simulink model "VSM_specComp_DC"  (R2024b)
settings: Solver=ode3  StartTime=0.0  StopTime=4  FixedStep=HWSampleTime  RelTol=1e-3
PostLoadFcn:
  | EXEC_MODE=ExecutionMode.SIMULATION;
  | %Sim_TP33_VSM_HSS_init
InitFcn:
  | %EXEC_MODE=ExecutionMode.SIMULATION;
  | %Sim_TP33_VSM_HSS_init
StopFcn:
  | %sim2struct
undefined symbols (not defined in the file): ControlSampleTime, DiscIntNeverNeededParam, fault_dur, Grid, HWSampleTime, Ion, LCL, Lithium, Manage, Param, SM, t_fault, V_DC, VSMCTRL
libraries: FriedrichLibrary x76, simulink x32, TriphaseHardwaremodule x24, spsThreePhaseSeriesRLCBranchLib x8, spsThreePhaseVIMeasurementLib x8, spsThreePhaseBreakerLib x8, spsGroundLib x4, spsUniversalBridgeLib x4, spsVoltageMeasurementLib x4, spsEdgeDetectorLib x4, spsMeanLib x4, simulink_extras x4
(part 6 of 10)

== system VSM_specComp_DC/VSM_3/VSM1/VSM/CONTROL/Virtual Circuit1 ==
  Param : Inport
  Reset : Inport  Port=2
  i_dq0 : Inport  Port=3
  Phi : Inport  Port=4
  Bus Selector : BusSelector  OutputSignals=R1,L1
  Bus Selector1 : BusSelector  OutputSignals=R1t,tauR,L1t,tauL
  Current Predictor : Subsystem  Commented=on
  L_Matrix : Gain  Gain=[0 -1 0;1 0 0; 0 0 0]
  L_Matrix1 : Gain  Gain=[0 -1 0;1 0 0; 0 0 0]
  PT1 : Subsystem  mask{K=1, Init=0, Ts=ControlSampleTime}
      mask prompts: K "Gain"; Init "Initial input"; Ts "Sample time"
      mask DialogControl DescGroupVar Prompt: PT1 discrete
      mask DialogControl DescTextVar Prompt: Simple discrete PT1
      mask Display:
      | text(0.5,0.5,get_param(gcb,'K'),'HorizontalAlignment','center','VerticalAlignment','Bottom')
      | text(0.5,0.5,'1 + s.tau','HorizontalAlignment','center','VerticalAlignment','Top')
      | plot([0.3 0.7],[0.5 0.5])
  PT2 : Subsystem  Commented=on  mask{K=1, Init=0, Ts=ControlSampleTime}
      mask prompts: K "Gain"; Init "Initial input"; Ts "Sample time"
      mask DialogControl DescGroupVar Prompt: PT1 discrete
      mask DialogControl DescTextVar Prompt: Simple discrete PT1
      mask Display:
      | text(0.5,0.5,get_param(gcb,'K'),'HorizontalAlignment','center','VerticalAlignment','Bottom')
      | text(0.5,0.5,'1 + s.tau','HorizontalAlignment','center','VerticalAlignment','Top')
      | plot([0.3 0.7],[0.5 0.5])
  "Param " : InportShadow
  Phi1 : InportShadow  Port=4
  Product : Product  Multiplication=Matrix(*)
  Product1 : Product  Multiplication=Matrix(*)
  Product2 : Product  Commented=on  Multiplication=Matrix(*)
  Product3 : Product  Multiplication=Matrix(*)
  R_Matrix : Gain  Gain=[1 0 0;0 1 0; 0 0 0]
  R_Matrix1 : Gain  Gain=[1 0 0;0 1 0; 0 0 0]
  Reset1 : InportShadow  Port=2
  Scope : Scope  NumInputPorts=2
  Scope1 : Scope
  Sum : Sum  Inputs=++|
  Sum1 : Sum  Inputs=++|
  Sum2 : Sum  Inputs=|++
  " u_dq0" : Outport
  wires:
  Product3/1 -> Scope/1
  Reset1/1 -> PT2/3(Reset)
  Reset/1 -> PT1/3(Reset)
  Phi1/1 -> PT2/4(Phi)
  PT1/1(Y) -> Product1/2
  Sum2/1 -> " u_dq0"/1
  Sum1/1 -> Sum2/2
  Product2/1 -> Sum1/2, Scope1/1
  PT2/1(Y) -> Product2/2
  L_Matrix1/1 -> Product2/1
  Bus Selector1/3 -> L_Matrix1/1  "<L1t>"
  Bus Selector1/2 -> PT1/2(tau)  "<tauR>"
  Bus Selector1/4 -> PT2/2(tau)  "<tauL>"
  Bus Selector1/1 -> R_Matrix1/1  "<R1t>"
  Product1/1 -> Sum1/1, Scope/2
  R_Matrix1/1 -> Product1/1
  Product/1 -> Sum2/1
  "Param "/1 -> Bus Selector1/1
  Sum/1 -> Product/1
  R_Matrix/1 -> Sum/2, Product3/1
  L_Matrix/1 -> Sum/1
  Bus Selector/2 -> L_Matrix/1  "<L1>"
  i_dq0/1 -> Product/2, Product3/2, PT1/1(U), PT2/1(U)
  Bus Selector/1 -> R_Matrix/1  "<R1>"
  Param/1 -> Bus Selector/1

== system VSM_specComp_DC/VSM_3/VSM1/VSM/CONTROL/active_damping ==
  enable_damp_dq : Inport
  Reset : Inport  Port=2
  u_dq0 : Inport  Port=3
  Phi : Inport  Port=4
  Bus Selector : BusSelector  OutputSignals=Damp_dq,Damp_dq,Damp_CM,OmLead,OmLag
  Integrator (inertia) : DiscreteIntegrator  gainval=1  ExternalReset=rising  InitialConditionSource=external  InitialCondition=1  SampleTime=ControlSampleTime  ICPrevOutput=DiscIntNeverNeededParam  ICPrevScaledInput=DiscIntNeverNeededParam
  Mux : Mux  Inputs=3
  Product{,1..3} (4 alike) : Product
  Sum : Sum  Inputs=|+-
  Sum2 : Sum  Inputs=++|
  Unit Delay2 : UnitDelay  InitialCondition=[0 0 0]  SampleTime=ControlSampleTime  HasFrameUpgradeWarning=on
  dq0->ab0 phi : FriedrichLibrary/Transformations/dq0->ab0 phi  SystemSampleTime=-1  VariantActivationTime=update diagram  AllowFlexibleInterface=on  Latency=0  AutoFrameSizeCalculation=off
  damp_dq0 : Outport  VectorParamsAs1DForOutWhenUnconnected=off
  wires:
  Bus Selector/5 -> Product3/2  "<OmLag>"
  Bus Selector/4 -> Product2/1  "<OmLead>"
  dq0->ab0 phi/1 -> Integrator (inertia)/3
  Unit Delay2/1 -> dq0->ab0 phi/1
  Reset/1 -> Integrator (inertia)/2
  Phi/1 -> dq0->ab0 phi/2
  Product1/1 -> damp_dq0/1
  Mux/1 -> Product/1, Product1/1  "enable"
  Product/1 -> Product2/2, Sum2/1
  u_dq0/1 -> Product/2
  Bus Selector/3 -> Mux/3  "<Damp_CM>"
  Bus Selector/2 -> Mux/2  "<Damp_dq>"
  Bus Selector/1 -> Mux/1  "<Damp_dq>"
  enable_damp_dq/1 -> Bus Selector/1
  Sum/1 -> Integrator (inertia)/1
  Sum2/1 -> Product1/2, Product3/1
  Product3/1 -> Sum/2
  Integrator (inertia)/1 -> Sum2/2, Unit Delay2/1
  Product2/1 -> Sum/1

== system VSM_specComp_DC/VSM_3/VSM1/VSM/CONTROL/dq0 to duty ==
  phi_rad : Inport
  u_dq0 : Inport  Port=2
  u_dc : Inport  Port=3
  Bias : Bias  Bias=Ctrl.PWM.tauT*Ctrl.PU.omegab  SaturateOnIntegerOverflow=off
  Bus Creator3 : BusCreator  Inputs=2
  Divide : Product  Inputs=*/
  Gain : Gain  Gain=eye(NrChannels,3)  Multiplication=Matrix(K*u)
  Modulation : FriedrichLibrary/Transformations/Modulation  Method=Sine Modulation  Ts=ControlSampleTime
  SMA : FriedrichLibrary/Discrete Stuff/SMA  n_samples=1/ControlSampleTime/100  init_out=0
  Saturation : Saturate  UpperLimit=inf  LowerLimit=1
  Signal Specification1 : SignalSpecification
  dq0->ab0 phi : FriedrichLibrary/Transformations/dq0->ab0 phi  SystemSampleTime=-1  VariantActivationTime=update diagram  AllowFlexibleInterface=on  Latency=0  AutoFrameSizeCalculation=off
  d : Outport  VectorParamsAs1DForOutWhenUnconnected=off
  pwmDiag : Outport  Port=2  VectorParamsAs1DForOutWhenUnconnected=off
  wires:
  SMA/1 -> Divide/2
  Saturation/1 -> SMA/1
  Signal Specification1/1 -> d/1
  Gain/1 -> Signal Specification1/1, Bus Creator3/1  "pwm"
  Bus Creator3/1 -> pwmDiag/1  "pwmDiag"
  u_dc/1 -> Saturation/1
  Bias/1 -> dq0->ab0 phi/2
  Modulation/1 -> Gain/1
  dq0->ab0 phi/1 -> Divide/1
  Divide/1 -> Modulation/1  "ab0 norm"
  u_dq0/1 -> dq0->ab0 phi/1
  phi_rad/1 -> Bias/1, Bus Creator3/2  "phi"

== system VSM_specComp_DC/VSM_3/VSM1/VSM/CONTROL/i_dq_ctrl ==
  note: PI Control
  note: Outrouting
  note: Inrouting
  Param : Inport
  enable_cc : Inport  Port=2
  sp_cc : Inport  Port=3
  ms_i_inv_dq : Inport  Port=4
  u_ff_dq : Inport  Port=5
  u_inv_dq : Inport  Port=6
  Enable : EnablePort  StatesWhenEnabling=reset
  Bus Creator2 : BusCreator  Inputs=4
  Bus Selector13 : BusSelector  OutputSignals=init_u_inv
  Constant : Constant
  Demux : Demux  Outputs=2
  From1 : From  Commented=on  GotoTag=initU
  Gain1 : Gain  Commented=on  Gain=Kff
  Gain2 : Gain  Gain=L_inv
  Gain4 : Gain  Gain=[0 -1;1 0]  Multiplication=Matrix(K*u)
  Gain5 : Gain  Commented=on  Gain=1-Kff
  Mux : Mux  Inputs=2
  PI : Subsystem
  Product : Product
  Product1 : Product
  Product2 : Product
  Scope : Scope  NumInputPorts=3
  Step : Step  Time=8  Before=1  After=0  SampleTime=0
  Sum1 : Sum  Inputs=+++
  Sum2 : Sum  Commented=on  Inputs=|+-
  Sum3 : Sum  Inputs=|+-
  Switch1 : Switch  Commented=on  Criteria=u2 > Threshold  SaturateOnIntegerOverflow=off  InputSameDT=off
  sp_u_inv_dq : Outport  VectorParamsAs1DForOutWhenUnconnected=off
  CCdiag : Outport  Port=2  VectorParamsAs1DForOutWhenUnconnected=off
  wires:
  PI/1(u) -> Sum1/1  "pi"
  Constant/1 -> Product1/2, Product2/2
  Demux/1 -> Product2/1
  Product2/1 -> Mux/1
  Product1/1 -> Mux/2
  Demux/2 -> Product1/1
  Mux/1 -> PI/1(di)
  ms_i_inv_dq/1 -> Gain4/1, Sum3/2, [i_dq]
  Product/1 -> [sp_u_dq], sp_u_inv_dq/1
  Gain5/1 -> Switch1/3
  u_ff_dq/1 -> Gain5/1, Gain1/1, PI/2(u0), Scope/2
  [i_dq] -> Bus Creator2/2  "i_dq"
  [sp_i_dq] -> Bus Creator2/1  "sp_i_dq"
  Bus Creator2/1 -> CCdiag/1
  [Enable] -> Bus Creator2/4  "enable_cc"
  enable_cc/1 -> [Enable]  "enable_cc"
  [sp_u_dq] -> Bus Creator2/3  "sp_u_dq"
  [Enable] -> Product/1
  Bus Selector13/1 -> [initU]  "<init_u_inv>"
  Param/1 -> Bus Selector13/1
  sp_cc/1 -> Sum3/1, [sp_i_dq]
  Sum3/1 -> Demux/1
  [Enable] -> PI/Enable
  u_inv_dq/1 -> Switch1/1
  Sum1/1 -> Product/2, Scope/1
  From1/1 -> Switch1/2
  Gain2/1 -> Sum2/2  "dq decouple"
  Gain4/1 -> Gain2/1
  Switch1/1 -> Sum2/1

== system VSM_specComp_DC/VSM_3/VSM1/VSM/MANAGEMENT/Subsystem1 ==
  In1 : Inport
  <i_inv_dq0> : Inport  Port=2
  <u_cap_ab0> : Inport  Port=3
  <PQ_out> : Inport  Port=4
  enable : Inport  Port=5
  "AL brechen AL nicht mit FCN lösbar " : Memory
  Add2 : Sum  Inputs=+-
  Constant : Constant
  Divide : Product  Inputs=*/
  Math Function1 : Math  Operator=square  SignedPower=on
  Math Function2 : Math  Operator=square  SignedPower=on
  Selector2 : Selector  InputPortWidth=3  IndexOptions=Index vector (dialog)  Indices=[1 2]  OutputSizes=1
  Sqrt1 : Sqrt
  Sqrt2 : Sqrt
  Subsystem : Subsystem
  Subsystem1 : Subsystem
  Sum of Elements1 : Sum  Inputs=+
  Sum of Elements2 : Sum  Inputs=+
  CC : Outport
  sp_CC : Outport  Port=2
  wires:
  Subsystem1/2(i_abs_pre) -> Subsystem/6(i abs_pre)
  Add2/1 -> Subsystem1/Enable
  enable/1 -> Subsystem/Enable, Add2/2
  Constant/1 -> Add2/1
  Divide/1 -> Subsystem1/1(In1)
  Subsystem1/1(i_pq_pre) -> Subsystem/5(PQ_pre)
  <PQ_out>/1 -> Subsystem/2(PQ_out), Divide/1
  Subsystem/2(CC) -> CC/1
  In1/1 -> Math Function1/1
  Subsystem/1(i_sp) -> sp_CC/1  "sp_CC"
  <i_inv_dq0>/1 -> "AL brechen AL nicht mit FCN lösbar "/1
  <u_cap_ab0>/1 -> Selector2/1
  Math Function2/1 -> Sum of Elements2/1
  Sqrt1/1 -> Subsystem/4(U_cap), Divide/2
  "AL brechen AL nicht mit FCN lösbar "/1 -> Subsystem/1(i_inv)
  Sum of Elements2/1 -> Sqrt1/1
  Sqrt2/1 -> Subsystem1/2(In2), Subsystem/3(iabs)
  Math Function1/1 -> Sum of Elements1/1
  Selector2/1 -> Math Function2/1
  Sum of Elements1/1 -> Sqrt2/1

== system VSM_specComp_DC/VSM_3/VSM1/VSM/MANAGEMENT/current_watchdog ==
  |i| set : Inport
  |i| reset : Inport  Port=2
  i_ab : Inport  Port=3
  sp_gain : Inport  Port=4
  PQ : Inport  Port=5
  i_inv : Inport  Port=6
  active_current_watchdog : EnablePort  StatesWhenEnabling=reset
  Divide : Product  Inputs=/**
  MATLAB Function : MATLAB Function  Commented=on  TreatAsAtomicUnit=on
  Math Function1 : Math  Operator=square  SignedPower=on
  Math Function2 : Math  Operator=square  SignedPower=on
  Math Function3 : Math  Operator=square  SignedPower=on
  Relational Operator : RelationalOperator  Operator=<=  OutDataTypeStr=boolean  InputSameDT=off
  Relational Operator1 : RelationalOperator  Operator=<=  OutDataTypeStr=boolean  InputSameDT=off
  S-R Flip-Flop1 : simulink_extras/Flip Flops/S-R Flip-Flop  initial_condition=0
  Scope : Scope  NumInputPorts=3
  Scope1 : Scope
  Sum of Elements1 : Sum  Inputs=+
  Terminator1 : Terminator
  enable_cc : Outport  VectorParamsAs1DForOutWhenUnconnected=off
  sp_gain_wd : Outport  Port=2  VectorParamsAs1DForOutWhenUnconnected=off
  wires:
  i_inv/1 -> MATLAB Function/4(i_inv)
  PQ/1 -> MATLAB Function/3(p), Scope1/1
  MATLAB Function/2(i) -> sp_gain_wd/1
  MATLAB Function/1(CC) -> Scope/1, enable_cc/1
  sp_gain/1 -> Divide/3
  |i| set/1 -> Math Function2/1, Divide/1
  |i| reset/1 -> Math Function3/1, Divide/2
  Math Function3/1 -> Relational Operator1/2
  S-R Flip-Flop1/2 -> Terminator1/1
  Relational Operator1/1 -> S-R Flip-Flop1/2
  Math Function1/1 -> Sum of Elements1/1
  Sum of Elements1/1 -> Relational Operator/2, MATLAB Function/1(abs), Relational Operator1/1
  i_ab/1 -> Math Function1/1
  Math Function2/1 -> MATLAB Function/2(set), Relational Operator/1

== system VSM_specComp_DC/VSM_3/VSM1/VSM/MANAGEMENT/sp_VSM ==
  EnableRateLimit : Inport
  CMD : Inport  Port=2
  MEAS : Inport  Port=3
  Bus Creator : BusCreator  Inputs=3
  Bus Selector1 : BusSelector  OutputSignals=u_out.u_out_ab0
  Bus Selector6 : BusSelector  OutputSignals=Param.VSM.sp_f,Param.VSM.sp_E,Param.VSM.sp_PQ,Param.VSM.sp_PQ_limit
  "CMD " : InportShadow  Port=2
  E(PQ) : Subsystem
  PQ(U) Limit : Subsystem
  RateLimit : Subsystem
  Saturation : Saturate  UpperLimit=1  LowerLimit=-1
  sp_VSM : Outport  VectorParamsAs1DForOutWhenUnconnected=off
  wires:
  Saturation/1 -> RateLimit/1(PQ)
  "CMD "/1 -> E(PQ)/2(cmd)
  Bus Creator/1 -> sp_VSM/1
  Bus Selector6/1 -> Bus Creator/1  "<sp_f>"
  MEAS/1 -> Bus Selector1/1
  CMD/1 -> Bus Selector6/1
  PQ(U) Limit/1(sp_PQ_limit) -> Bus Creator/3  "sp_PQ"
  Bus Selector6/4 -> PQ(U) Limit/2(enable)  "<sp_PQ_limit>"
  Bus Selector1/1 -> PQ(U) Limit/3(u_out)  "<u_out_ab0>"
  RateLimit/1(PQslow) -> PQ(U) Limit/1(sp_PQ), E(PQ)/3(sp_PQ)
  EnableRateLimit/1 -> RateLimit/Enable  "ENABLED"
  Bus Selector6/3 -> Saturation/1  "<sp_PQ>"
  Bus Selector6/2 -> E(PQ)/1(E)  "<sp_E>"
  E(PQ)/1(sp_E) -> Bus Creator/2  "sp_E"

== system VSM_specComp_DC/VSM_3/VSM1/VSM/Meas/SI -> pu ==
  MeasIn : Inport
  Bus Creator1 : BusCreator  Inputs=5
  Bus Selector : BusSelector  OutputSignals=meas_u_out,meas_i_out,meas_i_inverter,meas_u_dc,meas_u_cap
  Normalize : Gain  Gain=1/PU.Ub  OutDataTypeStr=double  RndMeth=Round
  Normalize1 : Gain  Gain=1/PU.Ib  OutDataTypeStr=double  RndMeth=Round
  Normalize2 : Gain  Gain=1/PU.Ib  OutDataTypeStr=double  RndMeth=Round
  Normalize3 : Gain  Gain=1/PU.Ub  OutDataTypeStr=double  RndMeth=Round
  Normalize4 : Gain  Gain=1/PU.Ub/2  OutDataTypeStr=double  RndMeth=Round
  MeasOut : Outport  VectorParamsAs1DForOutWhenUnconnected=off
  wires:
  MeasIn/1 -> Bus Selector/1
  Normalize/1 -> Bus Creator1/1  "meas_u_out"
  Normalize1/1 -> Bus Creator1/3  "meas_i_inverter"
  Normalize2/1 -> Bus Creator1/2  "meas_i_out"
  Normalize4/1 -> Bus Creator1/4  "meas_vol_dc"
  Bus Creator1/1 -> MeasOut/1
  Bus Selector/1 -> Normalize/1  "<meas_u_out>"
  Bus Selector/2 -> Normalize2/1  "<meas_i_out>"
  Bus Selector/3 -> Normalize1/1  "<meas_i_inverter>"
  Bus Selector/4 -> Normalize4/1  "<meas_u_dc>"
  Bus Selector/5 -> Normalize3/1  "<meas_u_cap>"
  Normalize3/1 -> Bus Creator1/5  "meas_u_cap"

== system VSM_specComp_DC/VSM_3/VSM1/VSM/Meas/meas_i_inv ==
  abc : Inport
  phi : Inport  Port=2
  Bus Creator1 : BusCreator  Inputs=3
  PhN->ab2 : FriedrichLibrary/Transformations/PhN->ab0  SystemSampleTime=-1  VariantActivationTime=update diagram  AllowFlexibleInterface=on  Latency=0  AutoFrameSizeCalculation=off
  ab0->dq0-faster : FriedrichLibrary/Transformations/ab0->dq0-faster  SystemSampleTime=-1  VariantActivationTime=update diagram  AllowFlexibleInterface=on  Latency=0  AutoFrameSizeCalculation=off
  i_inv_x : Outport  VectorParamsAs1DForOutWhenUnconnected=off
  wires:
  Bus Creator1/1 -> i_inv_x/1
  phi/1 -> ab0->dq0-faster/2
  abc/1 -> PhN->ab2/1, Bus Creator1/1  "i_inv_abc"
  PhN->ab2/1 -> ab0->dq0-faster/1, Bus Creator1/2  "i_inv_ab0"
  ab0->dq0-faster/1 -> Bus Creator1/3  "i_inv_dq0"

== system VSM_specComp_DC/VSM_3/VSM1/VSM/Meas/meas_i_out ==
  abc : Inport
  phi : Inport  Port=2
  Bus Creator1 : BusCreator  Inputs=3
  PhN->ab2 : FriedrichLibrary/Transformations/PhN->ab0  SystemSampleTime=-1  VariantActivationTime=update diagram  AllowFlexibleInterface=on  Latency=0  AutoFrameSizeCalculation=off
  ab0->dq0-faster : FriedrichLibrary/Transformations/ab0->dq0-faster  SystemSampleTime=-1  VariantActivationTime=update diagram  AllowFlexibleInterface=on  Latency=0  AutoFrameSizeCalculation=off
  i_out_x : Outport  VectorParamsAs1DForOutWhenUnconnected=off
  wires:
  Bus Creator1/1 -> i_out_x/1
  phi/1 -> ab0->dq0-faster/2
  abc/1 -> PhN->ab2/1, Bus Creator1/1  "i_out_abc"
  PhN->ab2/1 -> ab0->dq0-faster/1, Bus Creator1/2  "i_out_ab0"
  ab0->dq0-faster/1 -> Bus Creator1/3  "i_out_dq0"

== system VSM_specComp_DC/VSM_3/VSM1/VSM/Meas/meas_u_cap ==
  abc : Inport
  phi : Inport  Port=2
  Bus Creator1 : BusCreator  Inputs=3
  PhN->ab2 : FriedrichLibrary/Transformations/PhN->ab0  SystemSampleTime=-1  VariantActivationTime=update diagram  AllowFlexibleInterface=on  Latency=0  AutoFrameSizeCalculation=off
  ab0->dq0-faster : FriedrichLibrary/Transformations/ab0->dq0-faster  SystemSampleTime=-1  VariantActivationTime=update diagram  AllowFlexibleInterface=on  Latency=0  AutoFrameSizeCalculation=off
  u_cap_x : Outport  VectorParamsAs1DForOutWhenUnconnected=off
  wires:
  ab0->dq0-faster/1 -> Bus Creator1/3  "u_cap_dq0"
  PhN->ab2/1 -> Bus Creator1/2, ab0->dq0-faster/1  "u_cap_ab0"
  abc/1 -> Bus Creator1/1, PhN->ab2/1  "u_cap_abc"
  phi/1 -> ab0->dq0-faster/2
  Bus Creator1/1 -> u_cap_x/1

== system VSM_specComp_DC/VSM_3/VSM1/VSM/Meas/meas_u_out ==
  abc : Inport
  phi : Inport  Port=2
  Bus Creator1 : BusCreator  Inputs=3
  PhN->ab2 : FriedrichLibrary/Transformations/PhN->ab0  SystemSampleTime=-1  VariantActivationTime=update diagram  AllowFlexibleInterface=on  Latency=0  AutoFrameSizeCalculation=off
  ab0->dq0-faster : FriedrichLibrary/Transformations/ab0->dq0-faster  SystemSampleTime=-1  VariantActivationTime=update diagram  AllowFlexibleInterface=on  Latency=0  AutoFrameSizeCalculation=off
  u_out_x : Outport  VectorParamsAs1DForOutWhenUnconnected=off
  wires:
  ab0->dq0-faster/1 -> Bus Creator1/3  "u_out_dq0"
  PhN->ab2/1 -> Bus Creator1/2, ab0->dq0-faster/1  "u_out_ab0"
  abc/1 -> Bus Creator1/1, PhN->ab2/1  "u_out_abc"
  phi/1 -> ab0->dq0-faster/2
  Bus Creator1/1 -> u_out_x/1

== system VSM_specComp_DC/VSM_3/VSM1/command_center/cmd_VSM/Current Control ==
  note: else: init with u cap
  Bus Creator6 : BusCreator  Inputs=5
  Bus Creator7 : BusCreator  Inputs=3
  Init with u_inv [0/1] : Constant  Value=VSMCTRL.CC.init_uinv
  activate : Constant  Value=VSMCTRL.CC.activate
  external_stop_cc1 : Constant  Value=0
  external_stop_cc4 : Constant  Value=0
  i_reset_abs : Constant  Value=VSMCTRL.CC.i_reset
  i_set_abs : Constant  Value=VSMCTRL.CC.i_set
  i_sp_gain : Constant  Value=VSMCTRL.CC.i_sp_gain
  Current Control : Outport  VectorParamsAs1DForOutWhenUnconnected=off
  wires:
  Bus Creator6/1 -> Current Control/1  "CC"
  Init with u_inv [0/1]/1 -> Bus Creator6/1  "init_u_inv"
  external_stop_cc1/1 -> Bus Creator6/3  "ex_stop_cc"
  i_sp_gain/1 -> Bus Creator6/4  "i_sp_gain"
  i_set_abs/1 -> Bus Creator7/2  "abs_i_set"
  external_stop_cc4/1 -> Bus Creator6/2  "ex_start_cc"
  Bus Creator7/1 -> Bus Creator6/5  "watchdog"
  i_reset_abs/1 -> Bus Creator7/3  "abs_i_reset"
  activate/1 -> Bus Creator7/1  "activate"

== system VSM_specComp_DC/VSM_3/VSM1/command_center/cmd_VSM/Damping ==
  Bus Creator5 : BusCreator  Inputs=4
  EnableDamp_CM [0/1] : Constant  Value=VSMCTRL.VTFF.EnableCM
  EnableDamp_dq [0/1] : Constant  Value=VSMCTRL.VTFF.EnableDQ
  Omega Lag : Constant  Value=VSMCTRL.VTFF.OmLag
  Omega Lead : Constant  Value=VSMCTRL.VTFF.OmLead
  Damping : Outport  VectorParamsAs1DForOutWhenUnconnected=off
  wires:
  Omega Lag/1 -> Bus Creator5/4  "OmLag"
  Omega Lead/1 -> Bus Creator5/3  "OmLead"
  Bus Creator5/1 -> Damping/1
  EnableDamp_dq [0/1]/1 -> Bus Creator5/1  "Damp_dq"
  EnableDamp_CM [0/1]/1 -> Bus Creator5/2  "Damp_CM"

== system VSM_specComp_DC/VSM_3/VSM1/command_center/cmd_VSM/Manage ==
  Bus Creator : BusCreator  Inputs=2
  connect : Constant
  enable : Constant
  Manage : Outport  VectorParamsAs1DForOutWhenUnconnected=off
  wires:
  enable/1 -> Bus Creator/2  "enable"
  connect/1 -> Bus Creator/1  "connect"
  Bus Creator/1 -> Manage/1

== system VSM_specComp_DC/VSM_3/VSM1/command_center/cmd_VSM/Virtual Circuit ==
  Bus Creator9 : BusCreator  Inputs=7
  Virtual L1 : Constant  Value=VSMCTRL.VC.L1
  Virtual L1t : Constant  Value=VSMCTRL.VC.L1t
  Virtual R1 : Constant  Value=VSMCTRL.VC.R1
  Virtual R1t : Constant  Value=VSMCTRL.VC.R1t
  tau HP Slow : Constant  Value=VSMCTRL.VC.tauSlow
  tau Virtual L1 : Constant  Value=VSMCTRL.VC.tauL
  tau Virtual R1 : Constant  Value=VSMCTRL.VC.tauR
  Virtual Circuit : Outport  VectorParamsAs1DForOutWhenUnconnected=off
  wires:
  tau HP Slow/1 -> Bus Creator9/7  "tauS"
  tau Virtual L1/1 -> Bus Creator9/6  "tauL"
  tau Virtual R1/1 -> Bus Creator9/5  "tauR"
  Virtual L1/1 -> Bus Creator9/3  "L1"
  Bus Creator9/1 -> Virtual Circuit/1
  Virtual L1t/1 -> Bus Creator9/4  "L1t"
  Virtual R1t/1 -> Bus Creator9/2  "R1t"
  Virtual R1/1 -> Bus Creator9/1  "R1"

== system VSM_specComp_DC/VSM_3/VSM1/command_center/cmd_VSM/Virtual Synchronous Machine ==
  note: 0 Dekaktiviert Init Tiefpass
  note: 0 Dekaktiviert Init Tiefpass
  Bus Creator3 : BusCreator  Inputs=12
  E(sp_PQ) : Constant  Value=VSMCTRL.SP.E_comp
  Ta : Constant  Value=VSMCTRL.VSM.Ta
  Ta1 : Constant  Value=VSMCTRL.VSM.kpf
  Ta2 : Constant  Value=VSMCTRL.VSM.kdf
  Ta3 : Constant  Value=VSMCTRL.VSM.ku
  Ta4 : Constant  Value=VSMCTRL.VSM.Tu
  Ta5 : Constant  Value=0
  Ta6 : Constant  Value=0
  sp_E [pu] : Constant  Value=VSMCTRL.SP.E
  sp_PQ [pu] : Constant  Value=VSMCTRL.SP.PQ
  sp_PQ(U) limit : Constant  Value=VSMCTRL.SP.PQU_lim
  sp_f [Hz] : Constant  Value=VSMCTRL.SP.f
  Virtual Synchronous Machine : Outport  VectorParamsAs1DForOutWhenUnconnected=off
  wires:
  E(sp_PQ)/1 -> Bus Creator3/12  "sp_E_comp"
  Ta5/1 -> Bus Creator3/6  "Tuinit"
  Ta6/1 -> Bus Creator3/7  "TPinit"
  Ta1/1 -> Bus Creator3/2  "kpf"
  Ta2/1 -> Bus Creator3/3  "kdf"
  Ta3/1 -> Bus Creator3/4  "ku"
  Ta4/1 -> Bus Creator3/5  "Tu"
  Bus Creator3/1 -> Virtual Synchronous Machine/1
  Ta/1 -> Bus Creator3/1  "Ta"
  sp_PQ(U) limit/1 -> Bus Creator3/11  "sp_PQ_limit"
  sp_f [Hz]/1 -> Bus Creator3/8  "sp_f"
  sp_PQ [pu]/1 -> Bus Creator3/9  "sp_PQ"
  sp_E [pu]/1 -> Bus Creator3/10  "sp_E"

== system VSM_specComp_DC/VSM_4/VSM1/VSM/CONTROL/Subsystem1 ==
  <R1> : Inport
  <L1> : Inport  Port=2
  I : Inport  Port=3
  U_i : Inport  Port=4
  Enable : EnablePort
  MATLAB Function : MATLAB Function  TreatAsAtomicUnit=on
  Selector : Selector  InputPortWidth=3  IndexOptions=Index vector (dialog)  Indices=[1 2]  OutputSizes=1
  Selector1 : Selector  InputPortWidth=3  IndexOptions=Index vector (dialog)  Indices=[1 2]  OutputSizes=1
  phi_vsm : Outport
  U_v : Outport  Port=2
  wires:
  MATLAB Function/2(U_v) -> U_v/1
  MATLAB Function/1(phi_vsm) -> phi_vsm/1
  U_i/1 -> Selector1/1
  I/1 -> Selector/1
  Selector1/1 -> MATLAB Function/4(U_i)
  Selector/1 -> MATLAB Function/1(I)
  <R1>/1 -> MATLAB Function/3(R1)
  <L1>/1 -> MATLAB Function/2(L1)

== system VSM_specComp_DC/VSM_4/VSM1/VSM/CONTROL/VSMOC1 ==
  Manage : Inport
  Meas : Inport  Port=2
  u_inv_dq : Inport  Port=3
  Bus Selector1 : BusSelector  OutputSignals=enable_VSM.enable_ctrl,Param.VSM,enable_VSM.enable_inertia,sp_VSM
  Bus Selector11 : BusSelector  OutputSignals=phi
  Bus Selector2 : BusSelector  OutputSignals=PQ,PLL,u_cap.u_cap_dq0
  Selector : Selector  InputPortWidth=3  IndexOptions=Index vector (dialog)  Indices=[1 2]  OutputSizes=1
  Switch : Switch  Criteria=u2 ~= 0  SaturateOnIntegerOverflow=off  InputSameDT=off
  VSMOC : Subsystem
  phi_rad : Outport  VectorParamsAs1DForOutWhenUnconnected=off
  sp_u_inv_dq : Outport  Port=2  InitialOutput=[1 0]  VectorParamsAs1DForOutWhenUnconnected=off
  VSMdiag : Outport  Port=3  VectorParamsAs1DForOutWhenUnconnected=off
  wires:
  Bus Selector11/1 -> Switch/3  "<phi>"
  VSMOC/1(phi_rad) -> Switch/1
  VSMOC/3(VSMdiag) -> VSMdiag/1
  VSMOC/2(sp_u_inv_dq) -> sp_u_inv_dq/1
  Switch/1 -> phi_rad/1
  Manage/1 -> Bus Selector1/1
  Bus Selector1/1 -> VSMOC/Enable, Switch/2  "<enable_ctrl>"
  Meas/1 -> Bus Selector2/1
  Bus Selector2/2 -> VSMOC/5(PLL), Bus Selector11/1  "<PLL>"
  Bus Selector1/2 -> VSMOC/1(Param)  "<VSM>"
  Bus Selector1/3 -> VSMOC/2(enable_inertia)  "<enable_inertia>"
  Bus Selector1/4 -> VSMOC/3(sp_VSM)  "<sp_VSM>"
  u_inv_dq/1 -> VSMOC/6(u_inv_dq)
  Bus Selector2/3 -> Selector/1  "<u_cap_dq0>"
  Selector/1 -> VSMOC/7(u_cap_dq1)
  Bus Selector2/1 -> VSMOC/4(PQ_meas)  "<PQ>"

== system VSM_specComp_DC/VSM_4/VSM1/VSM/CONTROL/Virtual Circuit mit R und L ==
  Param : Inport
  Reset : Inport  Port=2
  i_dq0 : Inport  Port=3
  Phi : Inport  Port=4
  Bus Selector : BusSelector  OutputSignals=R1,L1
  Bus Selector1 : BusSelector  OutputSignals=R1t,tauR,L1t,tauL
  Current Predictor : Subsystem  Commented=on
  L_Matrix : Gain  Gain=[0 -1 0;1 0 0; 0 0 0]
  L_Matrix1 : Gain  Gain=[0 -1 0;1 0 0; 0 0 0]
  PT1 : Subsystem  mask{K=1, Init=0, Ts=ControlSampleTime}
      mask prompts: K "Gain"; Init "Initial input"; Ts "Sample time"
      mask DialogControl DescGroupVar Prompt: PT1 discrete
      mask DialogControl DescTextVar Prompt: Simple discrete PT1
      mask Display:
      | text(0.5,0.5,get_param(gcb,'K'),'HorizontalAlignment','center','VerticalAlignment','Bottom')
      | text(0.5,0.5,'1 + s.tau','HorizontalAlignment','center','VerticalAlignment','Top')
      | plot([0.3 0.7],[0.5 0.5])
  PT2 : Subsystem  mask{K=1, Init=0, Ts=ControlSampleTime}
      mask prompts: K "Gain"; Init "Initial input"; Ts "Sample time"
      mask DialogControl DescGroupVar Prompt: PT1 discrete
      mask DialogControl DescTextVar Prompt: Simple discrete PT1
      mask Display:
      | text(0.5,0.5,get_param(gcb,'K'),'HorizontalAlignment','center','VerticalAlignment','Bottom')
      | text(0.5,0.5,'1 + s.tau','HorizontalAlignment','center','VerticalAlignment','Top')
      | plot([0.3 0.7],[0.5 0.5])
  "Param " : InportShadow
  Phi1 : InportShadow  Port=4
  Product : Product  Multiplication=Matrix(*)
  Product1 : Product  Multiplication=Matrix(*)
  Product2 : Product  Multiplication=Matrix(*)
  R_Matrix : Gain  Gain=[1 0 0;0 1 0; 0 0 0]
  R_Matrix1 : Gain  Gain=[1 0 0;0 1 0; 0 0 0]
  Reset1 : InportShadow  Port=2
  Sum : Sum  Inputs=++|
  Sum1 : Sum  Inputs=++|
  Sum2 : Sum  Inputs=|++
  " u_dq0" : Outport
  wires:
  Param/1 -> Bus Selector/1
  Bus Selector/1 -> R_Matrix/1  "<R1>"
  i_dq0/1 -> Product/2, PT2/1(U), PT1/1(U)
  Bus Selector/2 -> L_Matrix/1  "<L1>"
  L_Matrix/1 -> Sum/1
  R_Matrix/1 -> Sum/2
  Sum/1 -> Product/1
  "Param "/1 -> Bus Selector1/1
  R_Matrix1/1 -> Product1/1
  Product1/1 -> Sum1/1
  Bus Selector1/1 -> R_Matrix1/1  "<R1t>"
  Bus Selector1/4 -> PT2/2(tau)  "<tauL>"
  Bus Selector1/2 -> PT1/2(tau)  "<tauR>"
  Bus Selector1/3 -> L_Matrix1/1  "<L1t>"
  L_Matrix1/1 -> Product2/1
  Product2/1 -> Sum1/2
  Sum2/1 -> " u_dq0"/1
  PT1/1(Y) -> Product1/2
  Phi/1 -> PT1/4(Phi)
  Phi1/1 -> PT2/4(Phi)
  Reset/1 -> PT1/3(Reset)
  Reset1/1 -> PT2/3(Reset)
  PT2/1(Y) -> Product2/2
  Product/1 -> Sum2/1

== system VSM_specComp_DC/VSM_4/VSM1/VSM/CONTROL/Virtual Circuit1 ==
  Param : Inport
  Reset : Inport  Port=2
  i_dq0 : Inport  Port=3
  Phi : Inport  Port=4
  Bus Selector : BusSelector  OutputSignals=R1,L1
  Bus Selector1 : BusSelector  OutputSignals=R1t,tauR,L1t,tauL
  Current Predictor : Subsystem  Commented=on
  L_Matrix : Gain  Gain=[0 -1 0;1 0 0; 0 0 0]
  L_Matrix1 : Gain  Gain=[0 -1 0;1 0 0; 0 0 0]
  PT1 : Subsystem  mask{K=1, Init=0, Ts=ControlSampleTime}
      mask prompts: K "Gain"; Init "Initial input"; Ts "Sample time"
      mask DialogControl DescGroupVar Prompt: PT1 discrete
      mask DialogControl DescTextVar Prompt: Simple discrete PT1
      mask Display:
      | text(0.5,0.5,get_param(gcb,'K'),'HorizontalAlignment','center','VerticalAlignment','Bottom')
      | text(0.5,0.5,'1 + s.tau','HorizontalAlignment','center','VerticalAlignment','Top')
      | plot([0.3 0.7],[0.5 0.5])
  PT2 : Subsystem  Commented=on  mask{K=1, Init=0, Ts=ControlSampleTime}
      mask prompts: K "Gain"; Init "Initial input"; Ts "Sample time"
      mask DialogControl DescGroupVar Prompt: PT1 discrete
      mask DialogControl DescTextVar Prompt: Simple discrete PT1
      mask Display:
      | text(0.5,0.5,get_param(gcb,'K'),'HorizontalAlignment','center','VerticalAlignment','Bottom')
      | text(0.5,0.5,'1 + s.tau','HorizontalAlignment','center','VerticalAlignment','Top')
      | plot([0.3 0.7],[0.5 0.5])
  "Param " : InportShadow
  Phi1 : InportShadow  Port=4
  Product : Product  Multiplication=Matrix(*)
  Product1 : Product  Multiplication=Matrix(*)
  Product2 : Product  Commented=on  Multiplication=Matrix(*)
  Product3 : Product  Multiplication=Matrix(*)
  R_Matrix : Gain  Gain=[1 0 0;0 1 0; 0 0 0]
  R_Matrix1 : Gain  Gain=[1 0 0;0 1 0; 0 0 0]
  Reset1 : InportShadow  Port=2
  Scope : Scope  NumInputPorts=2
  Scope1 : Scope
  Sum : Sum  Inputs=++|
  Sum1 : Sum  Inputs=++|
  Sum2 : Sum  Inputs=|++
  " u_dq0" : Outport
  wires:
  Param/1 -> Bus Selector/1
  Bus Selector/1 -> R_Matrix/1  "<R1>"
  i_dq0/1 -> PT2/1(U), PT1/1(U), Product3/2, Product/2
  Bus Selector/2 -> L_Matrix/1  "<L1>"
  L_Matrix/1 -> Sum/1
  R_Matrix/1 -> Product3/1, Sum/2
  Sum/1 -> Product/1
  "Param "/1 -> Bus Selector1/1
  Product/1 -> Sum2/1
  R_Matrix1/1 -> Product1/1
  Product1/1 -> Scope/2, Sum1/1
  Bus Selector1/1 -> R_Matrix1/1  "<R1t>"
  Bus Selector1/4 -> PT2/2(tau)  "<tauL>"
  Bus Selector1/2 -> PT1/2(tau)  "<tauR>"
  Bus Selector1/3 -> L_Matrix1/1  "<L1t>"
  L_Matrix1/1 -> Product2/1
  PT2/1(Y) -> Product2/2
  Product2/1 -> Scope1/1, Sum1/2
  Sum1/1 -> Sum2/2
  Sum2/1 -> " u_dq0"/1
  PT1/1(Y) -> Product1/2
  Phi1/1 -> PT2/4(Phi)
  Reset/1 -> PT1/3(Reset)
  Reset1/1 -> PT2/3(Reset)
  Product3/1 -> Scope/1

== system VSM_specComp_DC/VSM_4/VSM1/VSM/CONTROL/active_damping ==
  enable_damp_dq : Inport
  Reset : Inport  Port=2
  u_dq0 : Inport  Port=3
  Phi : Inport  Port=4
  Bus Selector : BusSelector  OutputSignals=Damp_dq,Damp_dq,Damp_CM,OmLead,OmLag
  Integrator (inertia) : DiscreteIntegrator  gainval=1  ExternalReset=rising  InitialConditionSource=external  InitialCondition=1  SampleTime=ControlSampleTime  ICPrevOutput=DiscIntNeverNeededParam  ICPrevScaledInput=DiscIntNeverNeededParam
  Mux : Mux  Inputs=3
  Product{,1..3} (4 alike) : Product
  Sum : Sum  Inputs=|+-
  Sum2 : Sum  Inputs=++|
  Unit Delay2 : UnitDelay  InitialCondition=[0 0 0]  SampleTime=ControlSampleTime  HasFrameUpgradeWarning=on
  dq0->ab0 phi : FriedrichLibrary/Transformations/dq0->ab0 phi  SystemSampleTime=-1  VariantActivationTime=update diagram  AllowFlexibleInterface=on  Latency=0  AutoFrameSizeCalculation=off
  damp_dq0 : Outport  VectorParamsAs1DForOutWhenUnconnected=off
  wires:
  Product2/1 -> Sum/1
  Integrator (inertia)/1 -> Unit Delay2/1, Sum2/2
  Product3/1 -> Sum/2
  Sum2/1 -> Product3/1, Product1/2
  Sum/1 -> Integrator (inertia)/1
  enable_damp_dq/1 -> Bus Selector/1
  Bus Selector/1 -> Mux/1  "<Damp_dq>"
  Bus Selector/2 -> Mux/2  "<Damp_dq>"
  Bus Selector/3 -> Mux/3  "<Damp_CM>"
  u_dq0/1 -> Product/2
  Product/1 -> Sum2/1, Product2/2
  Mux/1 -> Product1/1, Product/1  "enable"
  Product1/1 -> damp_dq0/1
  Phi/1 -> dq0->ab0 phi/2
  Reset/1 -> Integrator (inertia)/2
  Unit Delay2/1 -> dq0->ab0 phi/1
  dq0->ab0 phi/1 -> Integrator (inertia)/3
  Bus Selector/4 -> Product2/1  "<OmLead>"
  Bus Selector/5 -> Product3/2  "<OmLag>"

== system VSM_specComp_DC/VSM_4/VSM1/VSM/CONTROL/dq0 to duty ==
  phi_rad : Inport
  u_dq0 : Inport  Port=2
  u_dc : Inport  Port=3
  Bias : Bias  Bias=Ctrl.PWM.tauT*Ctrl.PU.omegab  SaturateOnIntegerOverflow=off
  Bus Creator3 : BusCreator  Inputs=2
  Divide : Product  Inputs=*/
  Gain : Gain  Gain=eye(NrChannels,3)  Multiplication=Matrix(K*u)
  Modulation : FriedrichLibrary/Transformations/Modulation  Method=Sine Modulation  Ts=ControlSampleTime
  SMA : FriedrichLibrary/Discrete Stuff/SMA  n_samples=1/ControlSampleTime/100  init_out=0
  Saturation : Saturate  UpperLimit=inf  LowerLimit=1
  Signal Specification1 : SignalSpecification
  dq0->ab0 phi : FriedrichLibrary/Transformations/dq0->ab0 phi  SystemSampleTime=-1  VariantActivationTime=update diagram  AllowFlexibleInterface=on  Latency=0  AutoFrameSizeCalculation=off
  d : Outport  VectorParamsAs1DForOutWhenUnconnected=off
  pwmDiag : Outport  Port=2  VectorParamsAs1DForOutWhenUnconnected=off
  wires:
  phi_rad/1 -> Bus Creator3/2, Bias/1  "phi"
  u_dq0/1 -> dq0->ab0 phi/1
  Divide/1 -> Modulation/1  "ab0 norm"
  dq0->ab0 phi/1 -> Divide/1
  Modulation/1 -> Gain/1
  Bias/1 -> dq0->ab0 phi/2
  u_dc/1 -> Saturation/1
  Bus Creator3/1 -> pwmDiag/1  "pwmDiag"
  Gain/1 -> Bus Creator3/1, Signal Specification1/1  "pwm"
  Signal Specification1/1 -> d/1
  Saturation/1 -> SMA/1
  SMA/1 -> Divide/2

== system VSM_specComp_DC/VSM_4/VSM1/VSM/CONTROL/i_dq_ctrl ==
  note: Inrouting
  note: Outrouting
  note: PI Control
  Param : Inport
  enable_cc : Inport  Port=2
  sp_cc : Inport  Port=3
  ms_i_inv_dq : Inport  Port=4
  u_ff_dq : Inport  Port=5
  u_inv_dq : Inport  Port=6
  Enable : EnablePort  StatesWhenEnabling=reset
  Bus Creator2 : BusCreator  Inputs=4
  Bus Selector13 : BusSelector  OutputSignals=init_u_inv
  Constant : Constant
  Demux : Demux  Outputs=2
  From1 : From  Commented=on  GotoTag=initU
  Gain1 : Gain  Commented=on  Gain=Kff
  Gain2 : Gain  Gain=L_inv
  Gain4 : Gain  Gain=[0 -1;1 0]  Multiplication=Matrix(K*u)
  Gain5 : Gain  Commented=on  Gain=1-Kff
  Mux : Mux  Inputs=2
  PI : Subsystem
  Product : Product
  Product1 : Product
  Product2 : Product
  Scope : Scope  NumInputPorts=3
  Step : Step  Time=8  Before=1  After=0  SampleTime=0
  Sum1 : Sum  Inputs=+++
  Sum2 : Sum  Commented=on  Inputs=|+-
  Sum3 : Sum  Inputs=|+-
  Switch1 : Switch  Commented=on  Criteria=u2 > Threshold  SaturateOnIntegerOverflow=off  InputSameDT=off
  sp_u_inv_dq : Outport  VectorParamsAs1DForOutWhenUnconnected=off
  CCdiag : Outport  Port=2  VectorParamsAs1DForOutWhenUnconnected=off
  wires:
  Switch1/1 -> Sum2/1
  Gain4/1 -> Gain2/1
  Gain2/1 -> Sum2/2  "dq decouple"
  From1/1 -> Switch1/2
  Sum1/1 -> Scope/1, Product/2
  u_inv_dq/1 -> Switch1/1
  [Enable] -> PI/Enable
  Sum3/1 -> Demux/1
  sp_cc/1 -> [sp_i_dq], Sum3/1
  Param/1 -> Bus Selector13/1
  Bus Selector13/1 -> [initU]  "<init_u_inv>"
  [Enable] -> Product/1
  [sp_u_dq] -> Bus Creator2/3  "sp_u_dq"
  enable_cc/1 -> [Enable]  "enable_cc"
  [Enable] -> Bus Creator2/4  "enable_cc"
  Bus Creator2/1 -> CCdiag/1
  [sp_i_dq] -> Bus Creator2/1  "sp_i_dq"
  [i_dq] -> Bus Creator2/2  "i_dq"
  u_ff_dq/1 -> Scope/2, PI/2(u0), Gain1/1, Gain5/1
  Gain5/1 -> Switch1/3
  Product/1 -> sp_u_inv_dq/1, [sp_u_dq]
  ms_i_inv_dq/1 -> [i_dq], Sum3/2, Gain4/1
  Mux/1 -> PI/1(di)
  Demux/2 -> Product1/1
  Product1/1 -> Mux/2
  Product2/1 -> Mux/1
  Demux/1 -> Product2/1
  Constant/1 -> Product2/2, Product1/2
  PI/1(u) -> Sum1/1  "pi"

== system VSM_specComp_DC/VSM_4/VSM1/VSM/MANAGEMENT/Subsystem1 ==
  In1 : Inport
  <i_inv_dq0> : Inport  Port=2
  <u_cap_ab0> : Inport  Port=3
  <PQ_out> : Inport  Port=4
  enable : Inport  Port=5
  "AL brechen AL nicht mit FCN lösbar " : Memory
  Add2 : Sum  Inputs=+-
  Constant : Constant
  Divide : Product  Inputs=*/
  Math Function1 : Math  Operator=square  SignedPower=on
  Math Function2 : Math  Operator=square  SignedPower=on
  Selector2 : Selector  InputPortWidth=3  IndexOptions=Index vector (dialog)  Indices=[1 2]  OutputSizes=1
  Sqrt1 : Sqrt
  Sqrt2 : Sqrt
  Subsystem : Subsystem
  Subsystem1 : Subsystem
  Sum of Elements1 : Sum  Inputs=+
  Sum of Elements2 : Sum  Inputs=+
  CC : Outport
  sp_CC : Outport  Port=2
  wires:
  Sum of Elements1/1 -> Sqrt2/1
  Selector2/1 -> Math Function2/1
  Math Function1/1 -> Sum of Elements1/1
  Sqrt2/1 -> Subsystem/3(iabs), Subsystem1/2(In2)
  Sum of Elements2/1 -> Sqrt1/1
  "AL brechen AL nicht mit FCN lösbar "/1 -> Subsystem/1(i_inv)
  Sqrt1/1 -> Divide/2, Subsystem/4(U_cap)
  Math Function2/1 -> Sum of Elements2/1
  <u_cap_ab0>/1 -> Selector2/1
  <i_inv_dq0>/1 -> "AL brechen AL nicht mit FCN lösbar "/1
  Subsystem/1(i_sp) -> sp_CC/1  "sp_CC"
  In1/1 -> Math Function1/1
  Subsystem/2(CC) -> CC/1
  <PQ_out>/1 -> Divide/1, Subsystem/2(PQ_out)
  Subsystem1/1(i_pq_pre) -> Subsystem/5(PQ_pre)
  Divide/1 -> Subsystem1/1(In1)
  Constant/1 -> Add2/1
  enable/1 -> Add2/2, Subsystem/Enable
  Add2/1 -> Subsystem1/Enable
  Subsystem1/2(i_abs_pre) -> Subsystem/6(i abs_pre)

== system VSM_specComp_DC/VSM_4/VSM1/VSM/MANAGEMENT/current_watchdog ==
  |i| set : Inport
  |i| reset : Inport  Port=2
  i_ab : Inport  Port=3
  sp_gain : Inport  Port=4
  PQ : Inport  Port=5
  i_inv : Inport  Port=6
  active_current_watchdog : EnablePort  StatesWhenEnabling=reset
  Divide : Product  Inputs=/**
  MATLAB Function : MATLAB Function  Commented=on  TreatAsAtomicUnit=on
  Math Function1 : Math  Operator=square  SignedPower=on
  Math Function2 : Math  Operator=square  SignedPower=on
  Math Function3 : Math  Operator=square  SignedPower=on
  Relational Operator : RelationalOperator  Operator=<=  OutDataTypeStr=boolean  InputSameDT=off
  Relational Operator1 : RelationalOperator  Operator=<=  OutDataTypeStr=boolean  InputSameDT=off
  S-R Flip-Flop1 : simulink_extras/Flip Flops/S-R Flip-Flop  initial_condition=0
  Scope : Scope  NumInputPorts=3
  Scope1 : Scope
  Sum of Elements1 : Sum  Inputs=+
  Terminator1 : Terminator
  enable_cc : Outport  VectorParamsAs1DForOutWhenUnconnected=off
  sp_gain_wd : Outport  Port=2  VectorParamsAs1DForOutWhenUnconnected=off
  wires:
  Math Function2/1 -> Relational Operator/1, MATLAB Function/2(set)
  i_ab/1 -> Math Function1/1
  Sum of Elements1/1 -> Relational Operator1/1, MATLAB Function/1(abs), Relational Operator/2
  Math Function1/1 -> Sum of Elements1/1
  Relational Operator1/1 -> S-R Flip-Flop1/2
  S-R Flip-Flop1/2 -> Terminator1/1
  Math Function3/1 -> Relational Operator1/2
  |i| reset/1 -> Divide/2, Math Function3/1
  |i| set/1 -> Divide/1, Math Function2/1
  sp_gain/1 -> Divide/3
  MATLAB Function/1(CC) -> enable_cc/1, Scope/1
  MATLAB Function/2(i) -> sp_gain_wd/1
  PQ/1 -> Scope1/1, MATLAB Function/3(p)
  i_inv/1 -> MATLAB Function/4(i_inv)

== system VSM_specComp_DC/VSM_4/VSM1/VSM/MANAGEMENT/sp_VSM ==
  EnableRateLimit : Inport
  CMD : Inport  Port=2
  MEAS : Inport  Port=3
  Bus Creator : BusCreator  Inputs=3
  Bus Selector1 : BusSelector  OutputSignals=u_out.u_out_ab0
  Bus Selector6 : BusSelector  OutputSignals=Param.VSM.sp_f,Param.VSM.sp_E,Param.VSM.sp_PQ,Param.VSM.sp_PQ_limit
  "CMD " : InportShadow  Port=2
  E(PQ) : Subsystem
  PQ(U) Limit : Subsystem
  RateLimit : Subsystem
  Saturation : Saturate  UpperLimit=1  LowerLimit=-1
  sp_VSM : Outport  VectorParamsAs1DForOutWhenUnconnected=off
  wires:
  E(PQ)/1(sp_E) -> Bus Creator/2  "sp_E"
  Bus Selector6/2 -> E(PQ)/1(E)  "<sp_E>"
  Bus Selector6/3 -> Saturation/1  "<sp_PQ>"
  EnableRateLimit/1 -> RateLimit/Enable  "ENABLED"
  RateLimit/1(PQslow) -> E(PQ)/3(sp_PQ), PQ(U) Limit/1(sp_PQ)
  Bus Selector1/1 -> PQ(U) Limit/3(u_out)  "<u_out_ab0>"
  Bus Selector6/4 -> PQ(U) Limit/2(enable)  "<sp_PQ_limit>"
  PQ(U) Limit/1(sp_PQ_limit) -> Bus Creator/3  "sp_PQ"
  CMD/1 -> Bus Selector6/1
  MEAS/1 -> Bus Selector1/1
  Bus Selector6/1 -> Bus Creator/1  "<sp_f>"
  Bus Creator/1 -> sp_VSM/1
  "CMD "/1 -> E(PQ)/2(cmd)
  Saturation/1 -> RateLimit/1(PQ)

== system VSM_specComp_DC/VSM_4/VSM1/VSM/Meas/SI -> pu ==
  MeasIn : Inport
  Bus Creator1 : BusCreator  Inputs=5
  Bus Selector : BusSelector  OutputSignals=meas_u_out,meas_i_out,meas_i_inverter,meas_u_dc,meas_u_cap
  Normalize : Gain  Gain=1/PU.Ub  OutDataTypeStr=double  RndMeth=Round
  Normalize1 : Gain  Gain=1/PU.Ib  OutDataTypeStr=double  RndMeth=Round
  Normalize2 : Gain  Gain=1/PU.Ib  OutDataTypeStr=double  RndMeth=Round
  Normalize3 : Gain  Gain=1/PU.Ub  OutDataTypeStr=double  RndMeth=Round
  Normalize4 : Gain  Gain=1/PU.Ub/2  OutDataTypeStr=double  RndMeth=Round
  MeasOut : Outport  VectorParamsAs1DForOutWhenUnconnected=off
  wires:
  Normalize3/1 -> Bus Creator1/5  "meas_u_cap"
  Bus Selector/5 -> Normalize3/1  "<meas_u_cap>"
  Bus Selector/4 -> Normalize4/1  "<meas_u_dc>"
  Bus Selector/3 -> Normalize1/1  "<meas_i_inverter>"
  Bus Selector/2 -> Normalize2/1  "<meas_i_out>"
  Bus Selector/1 -> Normalize/1  "<meas_u_out>"
  Bus Creator1/1 -> MeasOut/1
  Normalize4/1 -> Bus Creator1/4  "meas_vol_dc"
  Normalize2/1 -> Bus Creator1/2  "meas_i_out"
  Normalize1/1 -> Bus Creator1/3  "meas_i_inverter"
  Normalize/1 -> Bus Creator1/1  "meas_u_out"
  MeasIn/1 -> Bus Selector/1

== system VSM_specComp_DC/VSM_4/VSM1/VSM/Meas/meas_i_inv ==
  abc : Inport
  phi : Inport  Port=2
  Bus Creator1 : BusCreator  Inputs=3
  PhN->ab2 : FriedrichLibrary/Transformations/PhN->ab0  SystemSampleTime=-1  VariantActivationTime=update diagram  AllowFlexibleInterface=on  Latency=0  AutoFrameSizeCalculation=off
  ab0->dq0-faster : FriedrichLibrary/Transformations/ab0->dq0-faster  SystemSampleTime=-1  VariantActivationTime=update diagram  AllowFlexibleInterface=on  Latency=0  AutoFrameSizeCalculation=off
  i_inv_x : Outport  VectorParamsAs1DForOutWhenUnconnected=off
  wires:
  ab0->dq0-faster/1 -> Bus Creator1/3  "i_inv_dq0"
  PhN->ab2/1 -> Bus Creator1/2, ab0->dq0-faster/1  "i_inv_ab0"
  abc/1 -> Bus Creator1/1, PhN->ab2/1  "i_inv_abc"
  phi/1 -> ab0->dq0-faster/2
  Bus Creator1/1 -> i_inv_x/1

== system VSM_specComp_DC/VSM_4/VSM1/VSM/Meas/meas_i_out ==
  abc : Inport
  phi : Inport  Port=2
  Bus Creator1 : BusCreator  Inputs=3
  PhN->ab2 : FriedrichLibrary/Transformations/PhN->ab0  SystemSampleTime=-1  VariantActivationTime=update diagram  AllowFlexibleInterface=on  Latency=0  AutoFrameSizeCalculation=off
  ab0->dq0-faster : FriedrichLibrary/Transformations/ab0->dq0-faster  SystemSampleTime=-1  VariantActivationTime=update diagram  AllowFlexibleInterface=on  Latency=0  AutoFrameSizeCalculation=off
  i_out_x : Outport  VectorParamsAs1DForOutWhenUnconnected=off
  wires:
  ab0->dq0-faster/1 -> Bus Creator1/3  "i_out_dq0"
  PhN->ab2/1 -> Bus Creator1/2, ab0->dq0-faster/1  "i_out_ab0"
  abc/1 -> Bus Creator1/1, PhN->ab2/1  "i_out_abc"
  phi/1 -> ab0->dq0-faster/2
  Bus Creator1/1 -> i_out_x/1

== system VSM_specComp_DC/VSM_4/VSM1/VSM/Meas/meas_u_cap ==
  abc : Inport
  phi : Inport  Port=2
  Bus Creator1 : BusCreator  Inputs=3
  PhN->ab2 : FriedrichLibrary/Transformations/PhN->ab0  SystemSampleTime=-1  VariantActivationTime=update diagram  AllowFlexibleInterface=on  Latency=0  AutoFrameSizeCalculation=off
  ab0->dq0-faster : FriedrichLibrary/Transformations/ab0->dq0-faster  SystemSampleTime=-1  VariantActivationTime=update diagram  AllowFlexibleInterface=on  Latency=0  AutoFrameSizeCalculation=off
  u_cap_x : Outport  VectorParamsAs1DForOutWhenUnconnected=off
  wires:
  Bus Creator1/1 -> u_cap_x/1
  phi/1 -> ab0->dq0-faster/2
  abc/1 -> PhN->ab2/1, Bus Creator1/1  "u_cap_abc"
  PhN->ab2/1 -> ab0->dq0-faster/1, Bus Creator1/2  "u_cap_ab0"
  ab0->dq0-faster/1 -> Bus Creator1/3  "u_cap_dq0"

== system VSM_specComp_DC/VSM_4/VSM1/VSM/Meas/meas_u_out ==
  abc : Inport
  phi : Inport  Port=2
  Bus Creator1 : BusCreator  Inputs=3
  PhN->ab2 : FriedrichLibrary/Transformations/PhN->ab0  SystemSampleTime=-1  VariantActivationTime=update diagram  AllowFlexibleInterface=on  Latency=0  AutoFrameSizeCalculation=off
  ab0->dq0-faster : FriedrichLibrary/Transformations/ab0->dq0-faster  SystemSampleTime=-1  VariantActivationTime=update diagram  AllowFlexibleInterface=on  Latency=0  AutoFrameSizeCalculation=off
  u_out_x : Outport  VectorParamsAs1DForOutWhenUnconnected=off
  wires:
  Bus Creator1/1 -> u_out_x/1
  phi/1 -> ab0->dq0-faster/2
  abc/1 -> PhN->ab2/1, Bus Creator1/1  "u_out_abc"
  PhN->ab2/1 -> ab0->dq0-faster/1, Bus Creator1/2  "u_out_ab0"
  ab0->dq0-faster/1 -> Bus Creator1/3  "u_out_dq0"

== system VSM_specComp_DC/VSM_4/VSM1/command_center/cmd_VSM/Current Control ==
  note: else: init with u cap
  Bus Creator6 : BusCreator  Inputs=5
  Bus Creator7 : BusCreator  Inputs=3
  Init with u_inv [0/1] : Constant  Value=VSMCTRL.CC.init_uinv
  activate : Constant  Value=VSMCTRL.CC.activate
  external_stop_cc1 : Constant  Value=0
  external_stop_cc4 : Constant  Value=0
  i_reset_abs : Constant  Value=VSMCTRL.CC.i_reset
  i_set_abs : Constant  Value=VSMCTRL.CC.i_set
  i_sp_gain : Constant  Value=VSMCTRL.CC.i_sp_gain
  Current Control : Outport  VectorParamsAs1DForOutWhenUnconnected=off
  wires:
  activate/1 -> Bus Creator7/1  "activate"
  i_reset_abs/1 -> Bus Creator7/3  "abs_i_reset"
  Bus Creator7/1 -> Bus Creator6/5  "watchdog"
  external_stop_cc4/1 -> Bus Creator6/2  "ex_start_cc"
  i_set_abs/1 -> Bus Creator7/2  "abs_i_set"
  i_sp_gain/1 -> Bus Creator6/4  "i_sp_gain"
  external_stop_cc1/1 -> Bus Creator6/3  "ex_stop_cc"
  Init with u_inv [0/1]/1 -> Bus Creator6/1  "init_u_inv"
  Bus Creator6/1 -> Current Control/1  "CC"

== system VSM_specComp_DC/VSM_4/VSM1/command_center/cmd_VSM/Damping ==
  Bus Creator5 : BusCreator  Inputs=4
  EnableDamp_CM [0/1] : Constant  Value=VSMCTRL.VTFF.EnableCM
  EnableDamp_dq [0/1] : Constant  Value=VSMCTRL.VTFF.EnableDQ
  Omega Lag : Constant  Value=VSMCTRL.VTFF.OmLag
  Omega Lead : Constant  Value=VSMCTRL.VTFF.OmLead
  Damping : Outport  VectorParamsAs1DForOutWhenUnconnected=off
  wires:
  EnableDamp_CM [0/1]/1 -> Bus Creator5/2  "Damp_CM"
  EnableDamp_dq [0/1]/1 -> Bus Creator5/1  "Damp_dq"
  Bus Creator5/1 -> Damping/1
  Omega Lead/1 -> Bus Creator5/3  "OmLead"
  Omega Lag/1 -> Bus Creator5/4  "OmLag"

== system VSM_specComp_DC/VSM_4/VSM1/command_center/cmd_VSM/Manage ==
  Bus Creator : BusCreator  Inputs=2
  connect : Constant
  enable : Constant
  Manage : Outport  VectorParamsAs1DForOutWhenUnconnected=off
  wires:
  Bus Creator/1 -> Manage/1
  connect/1 -> Bus Creator/1  "connect"
  enable/1 -> Bus Creator/2  "enable"

== system VSM_specComp_DC/VSM_4/VSM1/command_center/cmd_VSM/Virtual Circuit ==
  Bus Creator9 : BusCreator  Inputs=7
  Virtual L1 : Constant  Value=VSMCTRL.VC.L1
  Virtual L1t : Constant  Value=VSMCTRL.VC.L1t
  Virtual R1 : Constant  Value=VSMCTRL.VC.R1
  Virtual R1t : Constant  Value=VSMCTRL.VC.R1t
  tau HP Slow : Constant  Value=VSMCTRL.VC.tauSlow
  tau Virtual L1 : Constant  Value=VSMCTRL.VC.tauL
  tau Virtual R1 : Constant  Value=VSMCTRL.VC.tauR
  Virtual Circuit : Outport  VectorParamsAs1DForOutWhenUnconnected=off
  wires:
  Virtual R1/1 -> Bus Creator9/1  "R1"
  Virtual R1t/1 -> Bus Creator9/2  "R1t"
  Virtual L1t/1 -> Bus Creator9/4  "L1t"
  Bus Creator9/1 -> Virtual Circuit/1
  Virtual L1/1 -> Bus Creator9/3  "L1"
  tau Virtual R1/1 -> Bus Creator9/5  "tauR"
  tau Virtual L1/1 -> Bus Creator9/6  "tauL"
  tau HP Slow/1 -> Bus Creator9/7  "tauS"

== system VSM_specComp_DC/VSM_4/VSM1/command_center/cmd_VSM/Virtual Synchronous Machine ==
  note: 0 Dekaktiviert Init Tiefpass
  note: 0 Dekaktiviert Init Tiefpass
  Bus Creator3 : BusCreator  Inputs=12
  E(sp_PQ) : Constant  Value=VSMCTRL.SP.E_comp
  Ta : Constant  Value=VSMCTRL.VSM.Ta
  Ta1 : Constant  Value=VSMCTRL.VSM.kpf
  Ta2 : Constant  Value=VSMCTRL.VSM.kdf
  Ta3 : Constant  Value=VSMCTRL.VSM.ku
  Ta4 : Constant  Value=VSMCTRL.VSM.Tu
  Ta5 : Constant  Value=0
  Ta6 : Constant  Value=0
  sp_E [pu] : Constant  Value=VSMCTRL.SP.E
  sp_PQ [pu] : Constant  Value=VSMCTRL.SP.PQ
  sp_PQ(U) limit : Constant  Value=VSMCTRL.SP.PQU_lim
  sp_f [Hz] : Constant  Value=VSMCTRL.SP.f
  Virtual Synchronous Machine : Outport  VectorParamsAs1DForOutWhenUnconnected=off
  wires:
  sp_E [pu]/1 -> Bus Creator3/10  "sp_E"
  sp_PQ [pu]/1 -> Bus Creator3/9  "sp_PQ"
  sp_f [Hz]/1 -> Bus Creator3/8  "sp_f"
  sp_PQ(U) limit/1 -> Bus Creator3/11  "sp_PQ_limit"
  Ta/1 -> Bus Creator3/1  "Ta"
  Bus Creator3/1 -> Virtual Synchronous Machine/1
  Ta4/1 -> Bus Creator3/5  "Tu"
  Ta3/1 -> Bus Creator3/4  "ku"
  Ta2/1 -> Bus Creator3/3  "kdf"
  Ta1/1 -> Bus Creator3/2  "kpf"
  Ta6/1 -> Bus Creator3/7  "TPinit"
  Ta5/1 -> Bus Creator3/6  "Tuinit"
  E(sp_PQ)/1 -> Bus Creator3/12  "sp_E_comp"
